simulink model "smd1_pi_graphics"  (R2020a)
settings: Solver=FixedStepAuto  StartTime=0.0  StopTime=500  FixedStep=0.001  RelTol=1e-3
model workspace (MAT data in the model file):
  Sig = Simulink.Signal
  Sig.DataType = 'auto'
  Sig.Dimensions = -1
  Sig.DimensionsMode = 'auto'
  Sig.Complexity = 'auto'
  Sig.SampleTime = -1
  Sig.SamplingMode = 'auto'
  b = 0.2
  k = 1
  m = 1
  u = 1
settings Model: EnablePacing=on  PacingRate=0.018000  Creator=bengt  LastModifiedBy=vivek vivian
settings DataIOCC: ReturnWorkspaceOutputs=off
settings DebuggingCC: ArithmeticOperatorsInVariantConditions=warning
settings SFSimCC: SimUseLocalCustomCode=off  CustomCodeUndefinedFunction=UseInterfaceOnly
settings RTWCC: RTWUseLocalCustomCode=off
settings CodeAppCC: StateflowObjectComments=on

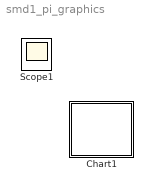
== system smd1_pi_graphics ==
  Chart1 : Stateflow chart  TreatAsAtomicUnit=on
  Scope1 : Scope

== stateflow chart smd1_pi_graphics/Chart1 ==
  settings: executeAtInitialization=1
  state Increment
    flag=1;
    en:x=x+0.1;y=y+0.1;
  state Wall1
    en:ml.move_mass(massH,x,y)
  state Start
    en: x=5;y=6;
    du: ml.move_mass(massH,x,y);
  state Top_Wall
    flag=0;
    en:x=x+0.1;y=y-0.1;
  state Wall2
    en:ml.move_mass(massH,x,y)
  state Right_Wall
    en:x=x+0.1;y=y+0.1;
  state Wall
    en:x=x-0.1;y=y+0.1;
  state Wall3
    en:ml.move_mass(massH,x,y)
  state Walll
    du:x=x-0.1;y=y-0.1;
  state Wall4
    en:ml.move_mass(massH,x,y)
  Increment -> Wall1 [order 2] : [y>=0]
  (default) -> Start : {ml.mk_fig();
      | axesH = ml.mk_axes();
      | massH = ml.mk_mass(axesH);}
  Start -> Increment
  Wall1 -> Increment [order 1] : [flag==1]
  Increment -> Top_Wall [order 1] : [y>=9.5]
  Top_Wall -> Wall1 [order 2] : {flag=0}
  Wall1 -> Top_Wall [order 2] : [x<19.5]
  Top_Wall -> Right_Wall [order 1] : [y<=0]
  Wall2 -> Right_Wall : [x<=19.5]
  Right_Wall -> Wall2 [order 1] : [x<=19.5]
  Right_Wall -> Wall [order 2] : [x>=19.5]
  Wall3 -> Wall
  Wall -> Wall3 [order 1] : [y<=9.5]
  Wall -> Walll [order 2] : [y>=9.5]
  Walll -> Wall4 : [x>0]
  Wall4 -> Walll
  data: massH local ml; axesH local ml; x local double; y local double; flag local double
